simulink model "main_spacecraft"  (R2023a)
settings: Solver=VariableStepAuto  StartTime=0.0  StopTime=Tfin  RelTol=1e-3
values from neighbouring files (symbols this model uses):
  K = nmpc_design_st2(par)    [ex1.m]
  r = [20 0 0 0 0 0]'    [ex1.m]
libraries: cstblocks x1
settings Model: Creator=marco  LastModifiedBy=marco

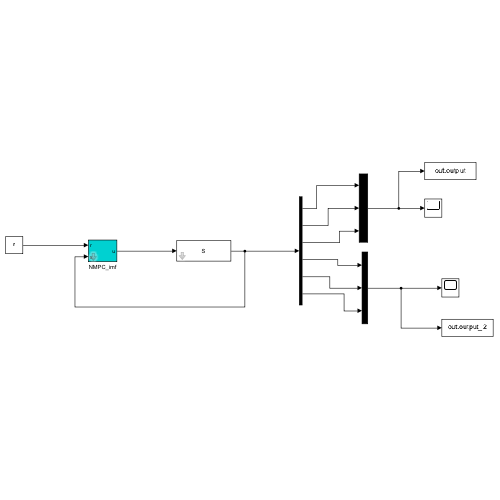
[thumbnail: Simulink's stored preview of the top-level diagram]
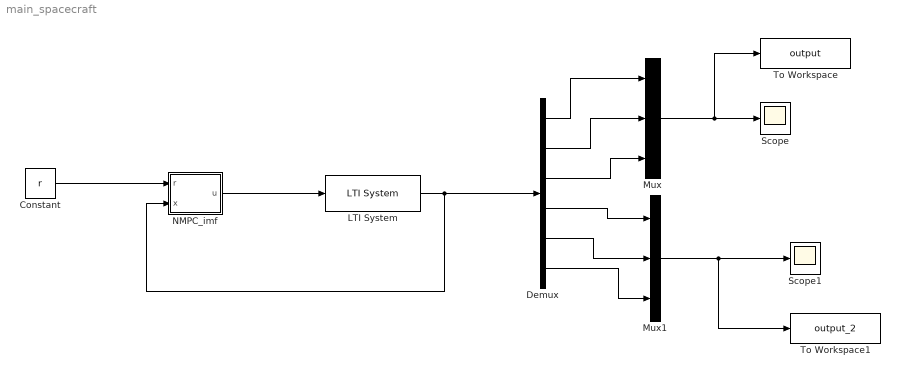
== system main_spacecraft ==
  Constant : Constant  Value=r
  Demux : Demux  Outputs=6
  LTI System : cstblocks/LTI System  sys=S  IC=x0
  Mux : Mux  Inputs=3
  Mux1 : Mux  Inputs=3
  NMPC_imf : Subsystem  mask{K=K}
      mask prompts: K "NMPC structure"
  Scope : Scope
  Scope1 : Scope
  To Workspace : ToWorkspace  VariableName=output  SaveFormat=Timeseries  SampleTime=-1
  To Workspace1 : ToWorkspace  VariableName=output_2  SaveFormat=Timeseries  SampleTime=-1
  wires:
  Constant/1 -> NMPC_imf/1(r)
  NMPC_imf/1(u) -> LTI System/1
  LTI System/1 -> Demux/1, NMPC_imf/2(x)
  Demux/4 -> Mux1/1
  Demux/5 -> Mux1/2
  Demux/6 -> Mux1/3
  Demux/1 -> Mux/1
  Demux/2 -> Mux/2
  Demux/3 -> Mux/3
  Mux1/1 -> To Workspace1/1, Scope1/1
  Mux/1 -> To Workspace/1, Scope/1

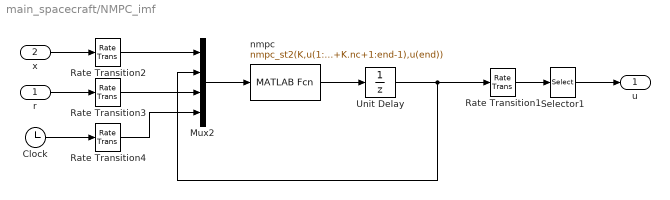
== system main_spacecraft/NMPC_imf ==
  r : Inport
  x : Inport  Port=2
  Clock : Clock
  Mux2 : Mux
  Rate Transition{1..4} (4 alike) : RateTransition  OutPortSampleTime=K.Ts
  Selector1 : Selector  InputPortWidth=K.nc  IndexOptions=Index vector (dialog)  Indices=1:K.nu  OutputSizes=1
  Unit Delay : UnitDelay  InitialCondition=zeros(K.nc,1)  SampleTime=K.Ts  HasFrameUpgradeWarning=on
  nmpc : MATLABFcn  MATLABFcn=nmpc_st2(K,u(1:K.nx),u(K.nx+1:K.nx+K.nc),u(K.nx+K.nc+1:end-1),u(end))  OutputDimensions=K.nc
  u : Outport  PortDimensions=K.nu
  wires:
  Rate Transition4/1 -> Mux2/4
  Clock/1 -> Rate Transition4/1
  Selector1/1 -> u/1
  nmpc/1 -> Unit Delay/1
  Rate Transition3/1 -> Mux2/3
  Rate Transition1/1 -> Selector1/1
  Rate Transition2/1 -> Mux2/1
  r/1 -> Rate Transition3/1
  Mux2/1 -> nmpc/1
  Unit Delay/1 -> Mux2/2, Rate Transition1/1
  x/1 -> Rate Transition2/1
